simulink model "ipm_foc_MTPA_fw"  (R2022b)
settings: Solver=VariableStepAuto  StartTime=0.0  StopTime=4  FixedStep=0.00001  RelTol=1e-4
values from neighbouring files (symbols this model uses):
  B = 0.00825    [im_params_fw.m]    (also in ipm_params_fw.m = 0.0005)
  Ismax = 6    [ipm_id_iq_wb.m]    (also in ipm_params_fw.m)
  J = 0.033    [im_params_fw.m]    (also in ipm_params_fw.m = 0.0002)
  Lamda_f = 0.272    [ipm_id_iq_wb.m]    (also in ipm_params_fw.m)
  Ld = 27e-3    (= 0.027)    [ipm_id_iq_wb.m]    (also in ipm_params_fw.m)
  Lq = 67e-3    (= 0.067)    [ipm_id_iq_wb.m]    (also in ipm_params_fw.m)
  pole = 4    [im_params_fw.m]    (also in ipm_params_fw.m)
  Rs = 0.8    [im_params_fw.m]    (also in ipm_params_fw.m = 4.3)
undefined symbols (not defined in the file or in its folder): sigbuilder_block
libraries: slpidlib x4
settings Model: Creator=jack  LastModifiedBy=jack
settings SolverCC: ZeroCrossAlgorithm=Adaptive
settings DebuggingCC: IgnoredZcDiagnostic=none

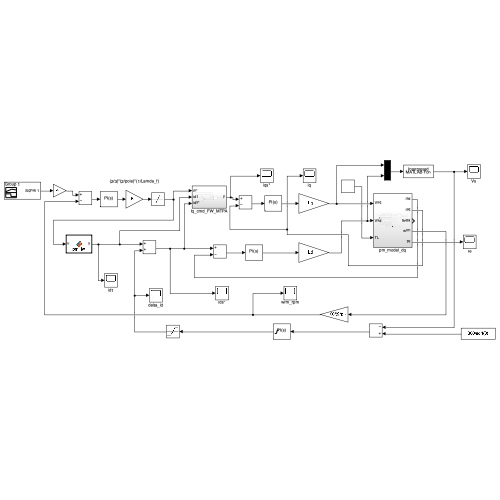
[thumbnail: Simulink's stored preview of the top-level diagram]
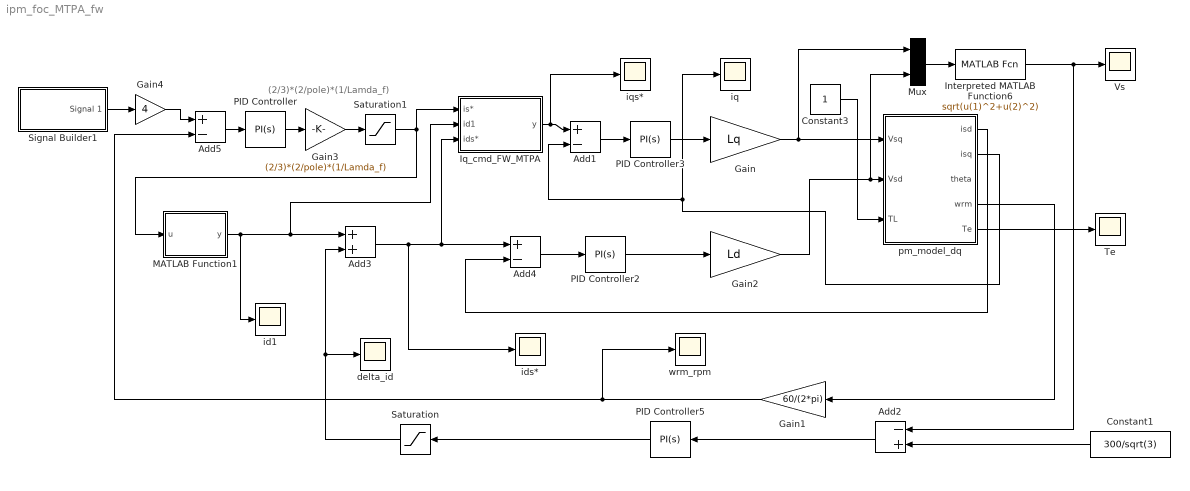
== system ipm_foc_MTPA_fw ==
  note: (2/3)*(2/pole)*(1/Lamda_f)
  Add1 : Sum  Inputs=+-
  Add2 : Sum  Inputs=-+
  Add3 : Sum
  Add4 : Sum  Inputs=+-
  Add5 : Sum  Inputs=+-
  Constant1 : Constant  Value=300/sqrt(3)
  Constant3 : Constant
  Gain : Gain  Gain=Lq
  Gain1 : Gain  Gain=60/(2*pi)
  Gain2 : Gain  Gain=Ld
  Gain3 : Gain  Gain=(2/3)*(2/pole)*(1/Lamda_f)
  Gain4 : Gain  Gain=4
  Interpreted MATLAB Function6 : MATLABFcn  MATLABFcn=sqrt(u(1)^2+u(2)^2)
  Iq_cmd_FW_MTPA : Subsystem
  MATLAB Function1 : MATLAB Function  TreatAsAtomicUnit=on
  Mux : Mux  Inputs=2
  PID Controller : slpidlib/PID Controller  Controller=PI  Form=Parallel  TimeDomain=Continuous-time  UseExternalTs=off  SampleTime=-1  IntegratorMethod=Forward Euler  FilterMethod=Forward Euler  ControllerParametersSource=internal  P=0.04  I=0.1  UseKiTs=off  D=0  N=100  UseFilter=on  TunerSelectOption=Transfer Function Based (PID Tuner App)  InitialConditionSource=internal  InitialConditionForIntegrator=0  InitialConditionForFilter=0  DifferentiatorICPrevScaledInput=0  ExternalReset=none  TrackingMode=off  Kt=1  LimitOutput=off  SatLimitsSource=internal  UpperSaturationLimit=inf  LowerSaturationLimit=-inf  LinearizeAsGain=on  AntiWindupMode=none  Kb=1  LimitIntegrator=off  UpperIntegratorSaturationLimit=inf  LowerIntegratorSaturationLimit=-inf  POutMin=[]  POutMax=[]  IOutMin=[]  IOutMax=[]  DOutMin=[]  DOutMax=[]  NOutMin=[]  NOutMax=[]  SumOutMin=[]  SumOutMax=[]  SaturationOutMin=[]  SaturationOutMax=[]  PParamMin=[]  PParamMax=[]  IParamMin=[]  IParamMax=[]  DParamMin=[]  DParamMax=[]  NParamMin=[]  NParamMax=[]  KbParamMin=[]  KbParamMax=[]  KtParamMin=[]  KtParamMax=[]  KbOutMin=[]  KbOutMax=[]  KtOutMin=[]  KtOutMax=[]  IntegratorOutMin=[]  IntegratorOutMax=[]  FilterOutMin=[]  FilterOutMax=[]  SumI1OutMin=[]  SumI1OutMax=[]  SumI2OutMin=[]  SumI2OutMax=[]  SumI3OutMin=[]  SumI3OutMax=[]  SumI4OutMin=[]  SumI4OutMax=[]  SumDOutMin=[]  SumDOutMax=[]  DifferentiatorOutMin=[]  DifferentiatorOutMax=[]  FilterDiffOutCoefMin=[]  FilterDiffOutCoefMax=[]  ReciprocalOutMin=[]  ReciprocalOutMax=[]  SumDenOutMin=[]  SumDenOutMax=[]  SumNumOutMin=[]  SumNumOutMax=[]  DivideOutMin=[]  DivideOutMax=[]  UdiffTsProdOutMin=[]  UdiffTsProdOutMax=[]  NTsProdOutMin=[]  NTsProdOutMax=[]  UintegralTsProdOutMin=[]  UintegralTsProdOutMax=[]  UngainTsProdOutMin=[]  UngainTsProdOutMax=[]  ClampingZeroOutDataTypeStr=Inherit: Inherit via back propagation  ClampingZeroOutMin=[]  ClampingZeroOutMax=[]  FilterDenConstantOutDataTypeStr=Inherit: Inherit via back propagation  FilterDenConstantOutMin=[]  FilterDenConstantOutMax=[]  PCopyOutDataTypeStr=Inherit: Inherit via back propagation  PCopyOutMin=[]  PCopyOutMax=[]  NCopyOutDataTypeStr=Inherit: Inherit via back propagation  NCopyOutMin=[]  NCopyOutMax=[]  IntegratorContinuousStateAttributes=''  IntegratorStateMustResolveToSignalObject=off  IntegratorRTWStateStorageClass=Auto  FilterContinuousStateAttributes=''  FilterStateMustResolveToSignalObject=off  FilterRTWStateStorageClass=Auto  ParallelPVariant=InternalParameters  IdealPVariant=Disabled  IVariant=InternalParameters  DVariant=Disabled  IntegratorVariant=Continuous  SatVariant=Disabled  AWVariant=Passthrough  PCopyVariant=Disabled  TRVariant=Disabled  FdbkBlocksVariant=Forward  IdealPFdbkVariant=Disabled  SatFdbkVariant=Disabled  DerivativeFilterVariant=Disabled  NVariant=Disabled  NCopyVariant=Disabled_SignalSpec  FilterICVariant=Disabled  IntegratorICVariant=InternalICs  ExternalResetVariant=Disabled  TRSumVariant=Passthrough  SumFdbkVariant=Disabled  SumVariant=Sum_PI  TsampFilterVariant=InternalTs  TsampNgainVariant=Passthrough  TsampIntegralVariant=Passthrough  ExternalSaturationOutDataTypeStr=Inherit: Same as second input
  PID Controller2 : slpidlib/PID Controller  Controller=PI  Form=Parallel  TimeDomain=Continuous-time  UseExternalTs=off  SampleTime=-1  IntegratorMethod=Forward Euler  FilterMethod=Forward Euler  ControllerParametersSource=internal  P=240  I=50000  UseKiTs=off  D=0  N=100  UseFilter=on  TunerSelectOption=Transfer Function Based (PID Tuner App)  InitialConditionSource=internal  InitialConditionForIntegrator=0  InitialConditionForFilter=0  DifferentiatorICPrevScaledInput=0  ExternalReset=none  TrackingMode=off  Kt=1  LimitOutput=off  SatLimitsSource=internal  UpperSaturationLimit=inf  LowerSaturationLimit=-inf  LinearizeAsGain=on  AntiWindupMode=none  Kb=1  LimitIntegrator=off  UpperIntegratorSaturationLimit=inf  LowerIntegratorSaturationLimit=-inf  POutMin=[]  POutMax=[]  IOutMin=[]  IOutMax=[]  DOutMin=[]  DOutMax=[]  NOutMin=[]  NOutMax=[]  SumOutMin=[]  SumOutMax=[]  SaturationOutMin=[]  SaturationOutMax=[]  PParamMin=[]  PParamMax=[]  IParamMin=[]  IParamMax=[]  DParamMin=[]  DParamMax=[]  NParamMin=[]  NParamMax=[]  KbParamMin=[]  KbParamMax=[]  KtParamMin=[]  KtParamMax=[]  KbOutMin=[]  KbOutMax=[]  KtOutMin=[]  KtOutMax=[]  IntegratorOutMin=[]  IntegratorOutMax=[]  FilterOutMin=[]  FilterOutMax=[]  SumI1OutMin=[]  SumI1OutMax=[]  SumI2OutMin=[]  SumI2OutMax=[]  SumI3OutMin=[]  SumI3OutMax=[]  SumI4OutMin=[]  SumI4OutMax=[]  SumDOutMin=[]  SumDOutMax=[]  DifferentiatorOutMin=[]  DifferentiatorOutMax=[]  FilterDiffOutCoefMin=[]  FilterDiffOutCoefMax=[]  ReciprocalOutMin=[]  ReciprocalOutMax=[]  SumDenOutMin=[]  SumDenOutMax=[]  SumNumOutMin=[]  SumNumOutMax=[]  DivideOutMin=[]  DivideOutMax=[]  UdiffTsProdOutMin=[]  UdiffTsProdOutMax=[]  NTsProdOutMin=[]  NTsProdOutMax=[]  UintegralTsProdOutMin=[]  UintegralTsProdOutMax=[]  UngainTsProdOutMin=[]  UngainTsProdOutMax=[]  ClampingZeroOutDataTypeStr=Inherit: Inherit via back propagation  ClampingZeroOutMin=[]  ClampingZeroOutMax=[]  FilterDenConstantOutDataTypeStr=Inherit: Inherit via back propagation  FilterDenConstantOutMin=[]  FilterDenConstantOutMax=[]  PCopyOutDataTypeStr=Inherit: Inherit via back propagation  PCopyOutMin=[]  PCopyOutMax=[]  NCopyOutDataTypeStr=Inherit: Inherit via back propagation  NCopyOutMin=[]  NCopyOutMax=[]  IntegratorContinuousStateAttributes=''  IntegratorStateMustResolveToSignalObject=off  IntegratorRTWStateStorageClass=Auto  FilterContinuousStateAttributes=''  FilterStateMustResolveToSignalObject=off  FilterRTWStateStorageClass=Auto  ParallelPVariant=InternalParameters  IdealPVariant=Disabled  IVariant=InternalParameters  DVariant=Disabled  IntegratorVariant=Continuous  SatVariant=Disabled  AWVariant=Passthrough  PCopyVariant=Disabled  TRVariant=Disabled  FdbkBlocksVariant=Forward  IdealPFdbkVariant=Disabled  SatFdbkVariant=Disabled  DerivativeFilterVariant=Disabled  NVariant=Disabled  NCopyVariant=Disabled_SignalSpec  FilterICVariant=Disabled  IntegratorICVariant=InternalICs  ExternalResetVariant=Disabled  TRSumVariant=Passthrough  SumFdbkVariant=Disabled  SumVariant=Sum_PI  TsampFilterVariant=InternalTs  TsampNgainVariant=Passthrough  TsampIntegralVariant=Passthrough  ExternalSaturationOutDataTypeStr=Inherit: Same as second input
  PID Controller3 : slpidlib/PID Controller  Controller=PI  Form=Parallel  TimeDomain=Continuous-time  UseExternalTs=off  SampleTime=-1  IntegratorMethod=Forward Euler  FilterMethod=Forward Euler  ControllerParametersSource=internal  P=2080  I=200000  UseKiTs=off  D=0  N=100  UseFilter=on  TunerSelectOption=Transfer Function Based (PID Tuner App)  InitialConditionSource=internal  InitialConditionForIntegrator=0  InitialConditionForFilter=0  DifferentiatorICPrevScaledInput=0  ExternalReset=none  TrackingMode=off  Kt=1  LimitOutput=off  SatLimitsSource=internal  UpperSaturationLimit=inf  LowerSaturationLimit=-inf  LinearizeAsGain=on  AntiWindupMode=none  Kb=1  LimitIntegrator=off  UpperIntegratorSaturationLimit=inf  LowerIntegratorSaturationLimit=-inf  POutMin=[]  POutMax=[]  IOutMin=[]  IOutMax=[]  DOutMin=[]  DOutMax=[]  NOutMin=[]  NOutMax=[]  SumOutMin=[]  SumOutMax=[]  SaturationOutMin=[]  SaturationOutMax=[]  PParamMin=[]  PParamMax=[]  IParamMin=[]  IParamMax=[]  DParamMin=[]  DParamMax=[]  NParamMin=[]  NParamMax=[]  KbParamMin=[]  KbParamMax=[]  KtParamMin=[]  KtParamMax=[]  KbOutMin=[]  KbOutMax=[]  KtOutMin=[]  KtOutMax=[]  IntegratorOutMin=[]  IntegratorOutMax=[]  FilterOutMin=[]  FilterOutMax=[]  SumI1OutMin=[]  SumI1OutMax=[]  SumI2OutMin=[]  SumI2OutMax=[]  SumI3OutMin=[]  SumI3OutMax=[]  SumI4OutMin=[]  SumI4OutMax=[]  SumDOutMin=[]  SumDOutMax=[]  DifferentiatorOutMin=[]  DifferentiatorOutMax=[]  FilterDiffOutCoefMin=[]  FilterDiffOutCoefMax=[]  ReciprocalOutMin=[]  ReciprocalOutMax=[]  SumDenOutMin=[]  SumDenOutMax=[]  SumNumOutMin=[]  SumNumOutMax=[]  DivideOutMin=[]  DivideOutMax=[]  UdiffTsProdOutMin=[]  UdiffTsProdOutMax=[]  NTsProdOutMin=[]  NTsProdOutMax=[]  UintegralTsProdOutMin=[]  UintegralTsProdOutMax=[]  UngainTsProdOutMin=[]  UngainTsProdOutMax=[]  ClampingZeroOutDataTypeStr=Inherit: Inherit via back propagation  ClampingZeroOutMin=[]  ClampingZeroOutMax=[]  FilterDenConstantOutDataTypeStr=Inherit: Inherit via back propagation  FilterDenConstantOutMin=[]  FilterDenConstantOutMax=[]  PCopyOutDataTypeStr=Inherit: Inherit via back propagation  PCopyOutMin=[]  PCopyOutMax=[]  NCopyOutDataTypeStr=Inherit: Inherit via back propagation  NCopyOutMin=[]  NCopyOutMax=[]  IntegratorContinuousStateAttributes=''  IntegratorStateMustResolveToSignalObject=off  IntegratorRTWStateStorageClass=Auto  FilterContinuousStateAttributes=''  FilterStateMustResolveToSignalObject=off  FilterRTWStateStorageClass=Auto  ParallelPVariant=InternalParameters  IdealPVariant=Disabled  IVariant=InternalParameters  DVariant=Disabled  IntegratorVariant=Continuous  SatVariant=Disabled  AWVariant=Passthrough  PCopyVariant=Disabled  TRVariant=Disabled  FdbkBlocksVariant=Forward  IdealPFdbkVariant=Disabled  SatFdbkVariant=Disabled  DerivativeFilterVariant=Disabled  NVariant=Disabled  NCopyVariant=Disabled_SignalSpec  FilterICVariant=Disabled  IntegratorICVariant=InternalICs  ExternalResetVariant=Disabled  TRSumVariant=Passthrough  SumFdbkVariant=Disabled  SumVariant=Sum_PI  TsampFilterVariant=InternalTs  TsampNgainVariant=Passthrough  TsampIntegralVariant=Passthrough  ExternalSaturationOutDataTypeStr=Inherit: Same as second input
  PID Controller5 : slpidlib/PID Controller  Controller=PI  Form=Parallel  TimeDomain=Continuous-time  UseExternalTs=off  SampleTime=-1  IntegratorMethod=Forward Euler  FilterMethod=Forward Euler  ControllerParametersSource=internal  P=0.1  I=1  UseKiTs=off  D=0  N=100  UseFilter=on  TunerSelectOption=Transfer Function Based (PID Tuner App)  InitialConditionSource=internal  InitialConditionForIntegrator=0  InitialConditionForFilter=0  DifferentiatorICPrevScaledInput=0  ExternalReset=none  TrackingMode=off  Kt=1  LimitOutput=on  SatLimitsSource=internal  UpperSaturationLimit=20  LowerSaturationLimit=-20  LinearizeAsGain=off  AntiWindupMode=clamping  Kb=1  LimitIntegrator=off  UpperIntegratorSaturationLimit=inf  LowerIntegratorSaturationLimit=-inf  POutMin=[]  POutMax=[]  IOutMin=[]  IOutMax=[]  DOutMin=[]  DOutMax=[]  NOutMin=[]  NOutMax=[]  SumOutMin=[]  SumOutMax=[]  SaturationOutMin=[]  SaturationOutMax=[]  PParamMin=[]  PParamMax=[]  IParamMin=[]  IParamMax=[]  DParamMin=[]  DParamMax=[]  NParamMin=[]  NParamMax=[]  KbParamMin=[]  KbParamMax=[]  KtParamMin=[]  KtParamMax=[]  KbOutMin=[]  KbOutMax=[]  KtOutMin=[]  KtOutMax=[]  IntegratorOutMin=[]  IntegratorOutMax=[]  FilterOutMin=[]  FilterOutMax=[]  SumI1OutMin=[]  SumI1OutMax=[]  SumI2OutMin=[]  SumI2OutMax=[]  SumI3OutMin=[]  SumI3OutMax=[]  SumI4OutMin=[]  SumI4OutMax=[]  SumDOutMin=[]  SumDOutMax=[]  DifferentiatorOutMin=[]  DifferentiatorOutMax=[]  FilterDiffOutCoefMin=[]  FilterDiffOutCoefMax=[]  ReciprocalOutMin=[]  ReciprocalOutMax=[]  SumDenOutMin=[]  SumDenOutMax=[]  SumNumOutMin=[]  SumNumOutMax=[]  DivideOutMin=[]  DivideOutMax=[]  UdiffTsProdOutMin=[]  UdiffTsProdOutMax=[]  NTsProdOutMin=[]  NTsProdOutMax=[]  UintegralTsProdOutMin=[]  UintegralTsProdOutMax=[]  UngainTsProdOutMin=[]  UngainTsProdOutMax=[]  ClampingZeroOutDataTypeStr=Inherit: Inherit via back propagation  ClampingZeroOutMin=[]  ClampingZeroOutMax=[]  FilterDenConstantOutDataTypeStr=Inherit: Inherit via back propagation  FilterDenConstantOutMin=[]  FilterDenConstantOutMax=[]  PCopyOutDataTypeStr=Inherit: Inherit via back propagation  PCopyOutMin=[]  PCopyOutMax=[]  NCopyOutDataTypeStr=Inherit: Inherit via back propagation  NCopyOutMin=[]  NCopyOutMax=[]  IntegratorContinuousStateAttributes=''  IntegratorStateMustResolveToSignalObject=off  IntegratorRTWStateStorageClass=Auto  FilterContinuousStateAttributes=''  FilterStateMustResolveToSignalObject=off  FilterRTWStateStorageClass=Auto  ParallelPVariant=InternalParameters  IdealPVariant=Disabled  IVariant=InternalParameters  DVariant=Disabled  IntegratorVariant=Continuous  SatVariant=Enabled  AWVariant=ContClampingParallel  PCopyVariant=Disabled  TRVariant=Disabled  FdbkBlocksVariant=Forward  IdealPFdbkVariant=Disabled  SatFdbkVariant=Disabled  DerivativeFilterVariant=Disabled  NVariant=Disabled  NCopyVariant=Disabled_SignalSpec  FilterICVariant=Disabled  IntegratorICVariant=InternalICs  ExternalResetVariant=Disabled  TRSumVariant=Passthrough  SumFdbkVariant=Disabled  SumVariant=Sum_PI  TsampFilterVariant=InternalTs  TsampNgainVariant=Passthrough  TsampIntegralVariant=Passthrough  ExternalSaturationOutDataTypeStr=Inherit: Same as second input
  Saturation : Saturate  UpperLimit=0  LowerLimit=-3.13
  Saturation1 : Saturate  UpperLimit=Ismax  LowerLimit=-Ismax
  Signal Builder1 : Subsystem  Tag=STV Subsys  LoadFcn=sigbuilder_block('load');  StartFcn=sigbuilder_block('start');  StopFcn=sigbuilder_block('stop');  ClipboardFcn=sigbuilder_block('clipboard');  mask(Sigbuilder block){tuvar=[0:10]}
      mask help: Simulink:masks:SigbuilderBlock_MD
      mask init:
      | if ~strcmp(get_param(bdroot(gcbh),'SimulationStatus'),'stopped') tuvar = sigbuilder_block('maskInit'); end
      settings: CopyFcn=sigbuilder_block('copy');  DeleteFcn=sigbuilder_block('delete');  ModelCloseFcn=sigbuilder_block('modelClose');  PreSaveFcn=sigbuilder_block('preSave');  PauseFcn=sigbuilder_block('pause');  ContinueFcn=sigbuilder_block('continue');  NameChangeFcn=sigbuilder_block('namechange');  OpenFcn=sigbuilder_block('open',[346 179 550 400 ]);  CloseFcn=sigbuilder_block('close');
      mask Display: plot(0, 0, 100, 100,[2, 2, 32, 32, 2], [68, 8, 8, 68, 68],[32, 2], [38, 38], [32, 19, 2],[53, 60, 44], [32, 17, 17, 2],[16, 16, 31, 31]);txt = getActiveGroup(gcbh);text(2, 100, txt,'verticalAlignment', 'top');
  Te : Scope
  Vs : Scope
  delta_id : Scope
  id1 : Scope
  ids* : Scope
  iq : Scope
  iqs* : Scope
  pm_model_dq : Subsystem
  wrm_rpm : Scope
  wires:
  PID Controller/1 -> Gain3/1
  Add1/1 -> PID Controller3/1
  Add4/1 -> PID Controller2/1
  Add5/1 -> PID Controller/1
  Signal Builder1/1(Signal 1) -> Gain4/1
  Gain1/1 -> Add5/2, wrm_rpm/1
  Gain/1 -> Mux/1, pm_model_dq/1(Vsq)
  pm_model_dq/2(isq) -> Add1/2, iq/1
  pm_model_dq/1(isd) -> Add4/2
  Gain2/1 -> Mux/2, pm_model_dq/2(Vsd)
  Constant3/1 -> pm_model_dq/3(TL)
  pm_model_dq/5(Te) -> Te/1
  pm_model_dq/4(wrm) -> Gain1/1
  PID Controller2/1 -> Gain2/1
  PID Controller3/1 -> Gain/1
  Gain3/1 -> Saturation1/1
  Interpreted MATLAB Function6/1 -> Vs/1, Add2/1
  Mux/1 -> Interpreted MATLAB Function6/1
  Gain4/1 -> Add5/1
  MATLAB Function1/1(y) -> id1/1, Iq_cmd_FW_MTPA/2(id1), Add3/1
  PID Controller5/1 -> Saturation/1
  Saturation/1 -> Add3/2, delta_id/1
  Add2/1 -> PID Controller5/1
  Constant1/1 -> Add2/2
  Add3/1 -> ids*/1, Iq_cmd_FW_MTPA/3(ids*), Add4/1
  Saturation1/1 -> Iq_cmd_FW_MTPA/1(is*), MATLAB Function1/1(u)
  Iq_cmd_FW_MTPA/1(y) -> iqs*/1, Add1/1

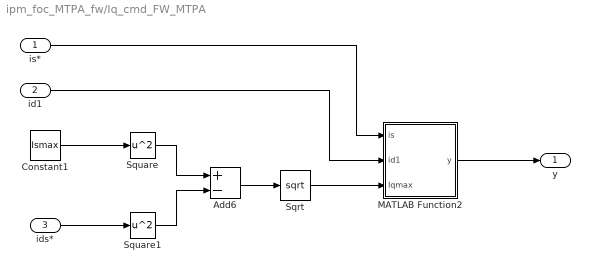
== system ipm_foc_MTPA_fw/Iq_cmd_FW_MTPA ==
  is* : Inport
  id1 : Inport  Port=2
  ids* : Inport  Port=3
  Add6 : Sum  Inputs=+-
  Constant1 : Constant  Value=Ismax
  MATLAB Function2 : MATLAB Function  TreatAsAtomicUnit=on
  Sqrt : Sqrt
  Square : Math  Operator=square
  Square1 : Math  Operator=square
  y : Outport
  wires:
  Square/1 -> Add6/1
  is*/1 -> MATLAB Function2/1(is)
  Square1/1 -> Add6/2
  Add6/1 -> Sqrt/1
  ids*/1 -> Square1/1
  MATLAB Function2/1(y) -> y/1
  Sqrt/1 -> MATLAB Function2/3(Iqmax)
  id1/1 -> MATLAB Function2/2(id1)
  Constant1/1 -> Square/1

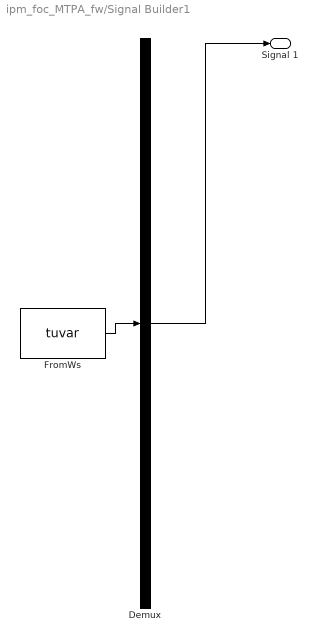
== system ipm_foc_MTPA_fw/Signal Builder1 ==
  Demux : Demux  Tag=STV Demux  Outputs=1
      settings: DisplayOption=none
  FromWs : FromWorkspace  Tag=STV FromWs  VariableName=tuvar
      SigBuilderData=|
      | common.afterFinalStr = 'Extrapolate'
      | common.sampleTime = 0
      | dataSet.timeRange = [0 10]
      | dataSet.name = 'Group 1'
      | sbobj.Groups.Name = 'Group 1'
      | sbobj.Groups.Signals.Name = 'Signal 1'
      | sbobj.Groups.Signals.XData = [0 1 4 6 10]
      | sbobj.Groups.Signals.YData = [0 1000 1000 1000 1000]
  Signal 1 : Outport  Tag=STV Outport
  wires:
  Demux/1 -> Signal 1/1
  FromWs/1 -> Demux/1

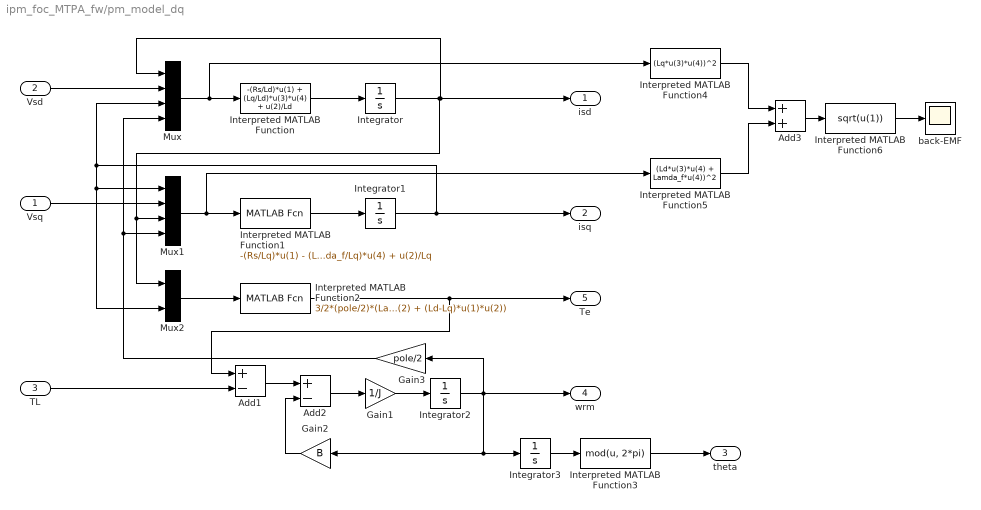
== system ipm_foc_MTPA_fw/pm_model_dq ==
  Vsq : Inport
  Vsd : Inport  Port=2
  TL : Inport  Port=3
  Add1 : Sum  Inputs=+-
  Add2 : Sum  Inputs=+-
  Add3 : Sum
  Gain1 : Gain  Gain=1/J
  Gain2 : Gain  Gain=B
  Gain3 : Gain  Gain=pole/2
  Integrator{,1..3} (4 alike) : Integrator
  Interpreted MATLAB Function : MATLABFcn  MATLABFcn=-(Rs/Ld)*u(1) + (Lq/Ld)*u(3)*u(4) + u(2)/Ld
  Interpreted MATLAB Function1 : MATLABFcn  MATLABFcn=-(Rs/Lq)*u(1) - (Ld/Lq)*u(3)*u(4) - (Lamda_f/Lq)*u(4) + u(2)/Lq
  Interpreted MATLAB Function2 : MATLABFcn  MATLABFcn=3/2*(pole/2)*(Lamda_f*u(2) + (Ld-Lq)*u(1)*u(2))
  Interpreted MATLAB Function3 : MATLABFcn  MATLABFcn=mod(u, 2*pi)
  Interpreted MATLAB Function4 : MATLABFcn  MATLABFcn=(Lq*u(3)*u(4))^2
  Interpreted MATLAB Function5 : MATLABFcn  MATLABFcn=(Ld*u(3)*u(4) + Lamda_f*u(4))^2
  Interpreted MATLAB Function6 : MATLABFcn  MATLABFcn=sqrt(u(1))
  Mux : Mux
  Mux1 : Mux
  Mux2 : Mux  Inputs=2
  back-EMF : Scope
  isd : Outport
  isq : Outport  Port=2
  theta : Outport  Port=3
  wrm : Outport  Port=4
  Te : Outport  Port=5
  wires:
  Mux/1 -> Interpreted MATLAB Function4/1, Interpreted MATLAB Function/1
  Interpreted MATLAB Function1/1 -> Integrator1/1
  TL/1 -> Add1/2
  Vsd/1 -> Mux/2
  Integrator1/1 -> isq/1, Mux/3, Mux2/2, Mux1/1
  Interpreted MATLAB Function2/1 -> Te/1, Add1/1
  Gain3/1 -> Mux/4, Mux1/4
  Add2/1 -> Gain1/1
  Gain1/1 -> Integrator2/1
  Add1/1 -> Add2/1
  Mux2/1 -> Interpreted MATLAB Function2/1
  Interpreted MATLAB Function/1 -> Integrator/1
  Vsq/1 -> Mux1/2
  Integrator/1 -> Mux2/1, Mux1/3, isd/1, Mux/1
  Integrator2/1 -> wrm/1, Gain3/1, Integrator3/1, Gain2/1
  Interpreted MATLAB Function3/1 -> theta/1
  Mux1/1 -> Interpreted MATLAB Function5/1, Interpreted MATLAB Function1/1
  Gain2/1 -> Add2/2
  Integrator3/1 -> Interpreted MATLAB Function3/1
  Add3/1 -> Interpreted MATLAB Function6/1
  Interpreted MATLAB Function5/1 -> Add3/2
  Interpreted MATLAB Function6/1 -> back-EMF/1
  Interpreted MATLAB Function4/1 -> Add3/1

== matlab function ipm_foc_MTPA_fw/MATLAB Function1 ==
  data: u input; y output
function y = pm_fw(u)
    Ld = 27e-3;
    Lq = 67e-3;
    Lamda_f = 0.272;
    y = (Lamda_f - sqrt(Lamda_f^2 + 8*(Lq-Ld)^2*u^2))/(4*(Lq-Ld));

== matlab function ipm_foc_MTPA_fw/Iq_cmd_FW_MTPA/MATLAB Function2 ==
  data: is input; y output; id1 input; Iqmax input
function y = iq_cmd(is, id1, Iqmax)
    iq1 = sqrt(is^2-id1^2);
    if (iq1 > Iqmax)
        y = Iqmax;
    elseif (iq1 < -Iqmax)
        y = -Iqmax;
    else
        y = iq1;
    end
